simulink model "SRM"  (R2025a)
settings: Solver=VariableStepAuto  StartTime=0.0  StopTime=2.00  RelTol=1e-3
values from neighbouring files (symbols this model uses):
  B = 0.001    [CODE.m]    (also in Controller.m = 0.0001; Moedl.m = Bmat; srm_mpc_setup.m = Bmat)
  Bp1_Current = linspace(0,180,181)    [Lut.m]    (also in Lut_1.m; Lut_Model.m)
  Bp2_Current = linspace(0,0.50,101)    [Lut.m]    (also in Lut_1.m = linspace(0,10,101); Lut_Model.m = linspace(0,10,101))
  J = 0.01    [CODE.m]    (also in Controller.m = 0.001; Lut.m; Moedl.m; srm_mpc_setup.m)
  LuT_Current = zeros(length(Bp1_Current), length(Bp2_Current))    [Lut.m]    (also in Lut_1.m; Lut_Model.m = zeros(181,101))
  Rs = 1    [CODE.m]    (also in Moedl.m; srm_mpc_setup.m)
libraries: spsDiodeLib x6, spsIGBTLib x6, spsVoltageMeasurementLib x3, spsDCVoltageSourceLib x1, sps_lib x1
settings Model: Creator=srima  LastModifiedBy=srima

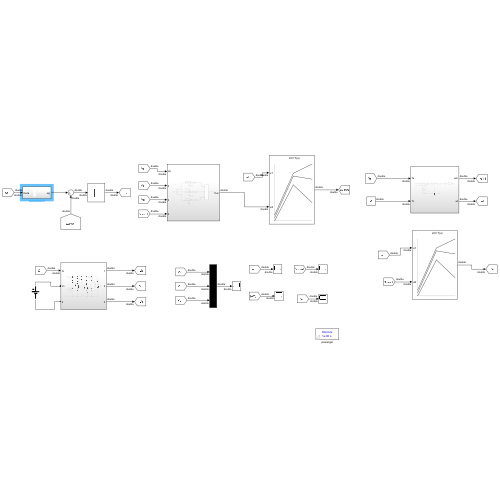
[thumbnail: Simulink's stored preview of the top-level diagram]
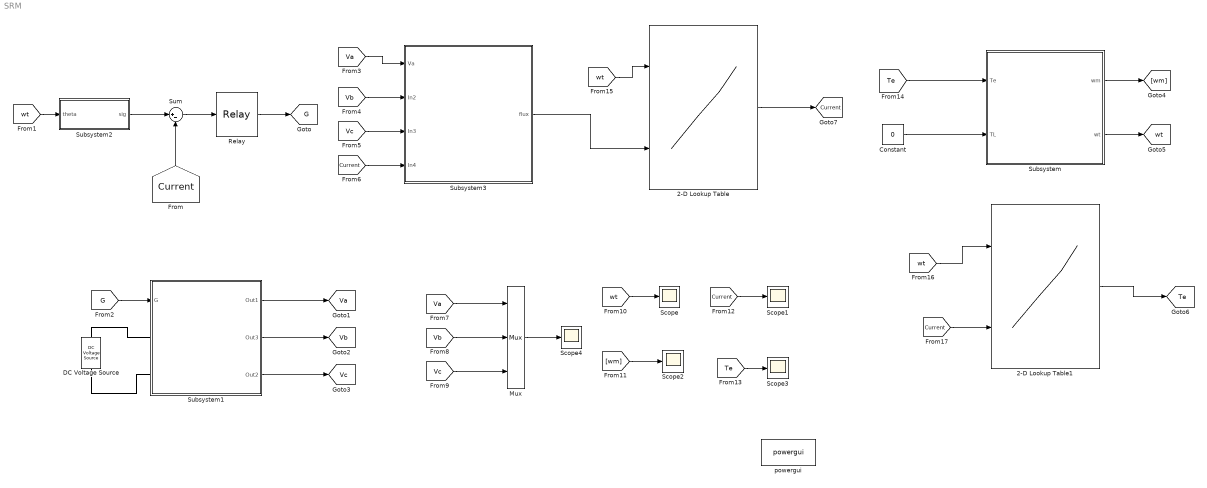
== system SRM ==
  2-D Lookup Table : Lookup_n-D  BreakpointsForDimension1=Bp1_Current  BreakpointsForDimension2=Bp2_Current  Table=LuT_Current  InternalRulePriority=Speed  RndMeth=Simplest
      settings: InputPortMap=u0,u1
  2-D Lookup Table1 : Lookup_n-D  BreakpointsForDimension1=Bp1_Current  BreakpointsForDimension2=Bp2_Current  Table=LuT_Current  InternalRulePriority=Speed  RndMeth=Simplest
      settings: InputPortMap=u0,u1
  Constant : Constant  Value=0
  DC Voltage Source : spsDCVoltageSourceLib/DC Voltage Source  Amplitude=240  Measurements=None
  Mux : Mux  Inputs=3
  Relay : Relay  OnSwitchValue=10  OffSwitchValue=-10
  Scope{,1..4} (5 alike) : Scope
      Scope settings: ActiveDisplayYMinimum=-13.273484846616352  ActiveDisplayYMaximum=186.28058756716342
      Scope1 settings: ActiveDisplayYMinimum=-525.72659240641281  ActiveDisplayYMaximum=1323.506067242982
      Scope2 settings: ActiveDisplayYMinimum=-1.6002807038142943E+8  ActiveDisplayYMaximum=2.6802963440797266E+8  DataLoggingVariableName=ScopeData2
      Scope3 settings: ActiveDisplayYMinimum=41724.804742170025  ActiveDisplayYMaximum=41770.999218996563  DataLoggingVariableName=ScopeData3
      Scope4 settings: ActiveDisplayYMinimum=-1  ActiveDisplayYMaximum=1  DataLoggingVariableName=ScopeData4
  Subsystem : Subsystem
  Subsystem1 : Subsystem
  Subsystem2 : Subsystem
  Subsystem3 : Subsystem
  Sum : Sum  Inputs=|+-
  powergui : sps_lib/powergui  Priority=1  SimulationMode=Discrete  SampleTime=1e-06  frequency=60  Iterations=50  frequencyindice=0  Pbase=100e6  ErrMax=1e-4  UnitsV=kV  UnitsW=MW  buscounter=0  FunctionMessages=off  echomessages=off  EnableUseOfTLC=off  CurrentSourceSwitches=off  DisableSnubberDevices=off  DisableRonSwitches=off  DisableVfSwitches=off  DisplayEquations=off  AutomaticDiscreteSolvers=off  SolverType=Tustin/Backward Euler (TBE)  Interpol=off  ExternalGateDelay=off  methode=off  Ts=100  x0status=blocks  SPID=on  SwTol=0  HookPort=off  NonlinearTolerance=1e-4  nMaxIteration=100  ContinueOnMaxIteration=off  RestoreLinks=warning  ResistiveCurrentMeasurement=off  Frange=[0:2:500]  Ylog=off  Xlog=on  ShowGrid=off  save=off  variable=ZData  structure=0  ZoomFFT=off  StartTime=0.0  cycles=1  DisplayStyle=1  fundamental=60  FreqAxis=off  MaxFrequency=1000  frequencyindicesteady=1  RmsSteady=1  display=off
  tag scope: Current=global, G=global, Te=global, Va=global, Vb=global, Vc=global, wt=global
  wires:
  Sum/1 -> Relay/1
  [Current] -> Sum/2
  Subsystem2/1(sig) -> Sum/1
  [wt] -> Subsystem2/1(theta)
  Relay/1 -> [G]
  Subsystem1/1(Out1) -> [Va]
  Subsystem1/2(Out3) -> [Vb]
  Subsystem1/3(Out2) -> [Vc]
  [G] -> Subsystem1/1(G)
  [Va] -> Subsystem3/1(Va)
  [Vb] -> Subsystem3/2(In2)
  [Vc] -> Subsystem3/3(In3)
  [Current] -> Subsystem3/4(In4)
  [Va] -> Mux/1
  [Vb] -> Mux/2
  [Vc] -> Mux/3
  Mux/1 -> Scope4/1
  [wt] -> Scope/1
  [wm] -> Scope2/1
  [Current] -> Scope1/1
  [Te] -> Scope3/1
  [Te] -> Subsystem/1(Te)
  Constant/1 -> Subsystem/2(TL)
  Subsystem/1(wm) -> [wm]
  Subsystem/2(wt) -> [wt]
  [wt] -> 2-D Lookup Table/1
  Subsystem3/1(flux) -> 2-D Lookup Table/2
  [wt] -> 2-D Lookup Table1/1
  [Current] -> 2-D Lookup Table1/2
  2-D Lookup Table1/1 -> [Te]
  2-D Lookup Table/1 -> [Current]
  connections:
  DC Voltage Source/RConn1 -- Subsystem1/LConn1
  DC Voltage Source/LConn1 -- Subsystem1/LConn2

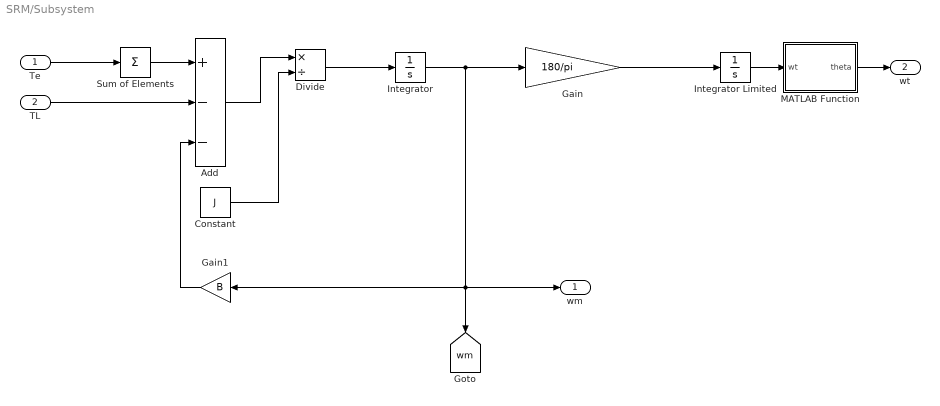
== system SRM/Subsystem ==
  Te : Inport
  TL : Inport  Port=2
  Add : Sum  Inputs=+--
  Constant : Constant  Value=J
  Divide : Product  Inputs=*/
  Gain : Gain  Gain=180/pi
  Gain1 : Gain  Gain=B
  Integrator : Integrator
  Integrator Limited : Integrator  InitialCondition=[0,30,60]  LimitOutput=on
  MATLAB Function : MATLAB Function  TreatAsAtomicUnit=on
  Sum of Elements : Sum  Inputs=+
  wm : Outport
  wt : Outport  Port=2
  tag scope: wm=global
  wires:
  Te/1 -> Sum of Elements/1
  Sum of Elements/1 -> Add/1
  TL/1 -> Add/2
  Gain1/1 -> Add/3
  Divide/1 -> Integrator/1
  Add/1 -> Divide/1
  Constant/1 -> Divide/2
  Gain/1 -> Integrator Limited/1
  Integrator/1 -> wm/1, [wm], Gain1/1, Gain/1
  MATLAB Function/1(theta) -> wt/1
  Integrator Limited/1 -> MATLAB Function/1(wt)

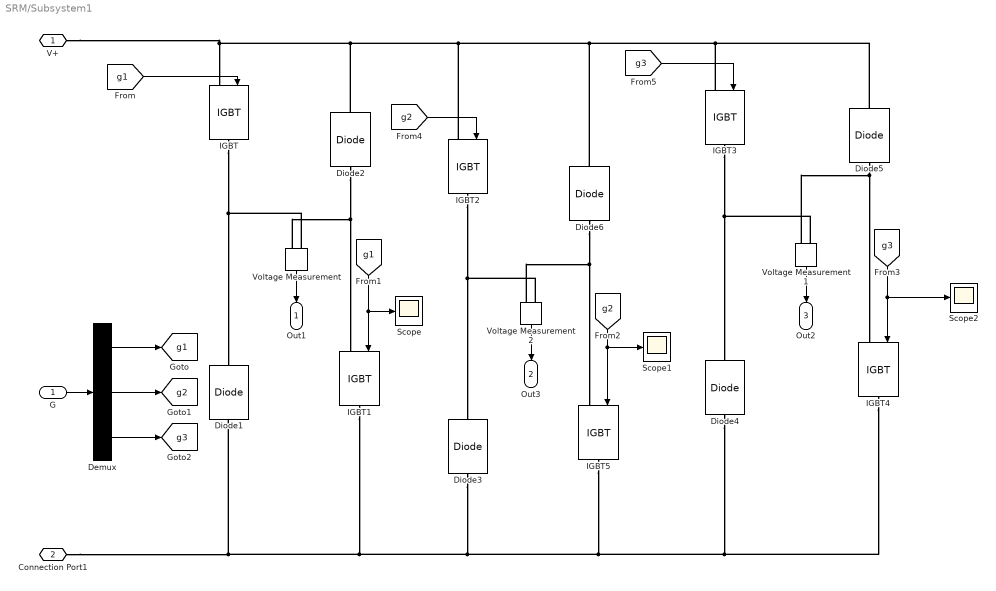
== system SRM/Subsystem1 ==
  G : Inport
  Demux : Demux  Outputs=3
  Diode1 : spsDiodeLib/Diode  Ron=1e-3  Lon=0  Vf=0.8  IC=0  UseSnubber=0  Rs=1000  Cs=inf  Measurements=off
  Diode2 : spsDiodeLib/Diode  Ron=0.001  Lon=0  Vf=0.8  IC=0  UseSnubber=0  Rs=500  Cs=250e-9  Measurements=off
  Diode3 : spsDiodeLib/Diode  Ron=1e-3  Lon=0  Vf=0.8  IC=0  UseSnubber=0  Rs=1000  Cs=inf  Measurements=off
  Diode4 : spsDiodeLib/Diode  Ron=1e-3  Lon=0  Vf=0.8  IC=0  UseSnubber=0  Rs=1000  Cs=inf  Measurements=off
  Diode5 : spsDiodeLib/Diode  Ron=0.001  Lon=0  Vf=0.8  IC=0  UseSnubber=0  Rs=500  Cs=250e-9  Measurements=off
  Diode6 : spsDiodeLib/Diode  Ron=0.001  Lon=0  Vf=0.8  IC=0  UseSnubber=0  Rs=500  Cs=250e-9  Measurements=off
  IGBT{,1..5} (6 alike) : spsIGBTLib/IGBT  Ron=0.001  Lon=0  Vf=1  Tf=1e-6  Tt=2e-6  IC=0  Rs=1e5  Cs=inf  Measurements=off
  Scope : Scope
      settings: ActiveDisplayYMinimum=-0.37134694290744508  ActiveDisplayYMaximum=1.3037726078738059  DataLoggingVariableName=ScopeData5
  Scope1 : Scope
      settings: ActiveDisplayYMinimum=-0.72000513153914225  ActiveDisplayYMaximum=1.7549093677601073  DataLoggingVariableName=ScopeData6
  Scope2 : Scope
      settings: ActiveDisplayYMinimum=-0.70342994389969249  ActiveDisplayYMaximum=5.381855163203106  DataLoggingVariableName=ScopeData7
  Voltage Measurement : spsVoltageMeasurementLib/Voltage Measurement  PhasorSimulation=off  OutputType=Complex  PSBequivalent=0
  Voltage Measurement1 : spsVoltageMeasurementLib/Voltage Measurement  PhasorSimulation=off  OutputType=Complex  PSBequivalent=0
  Voltage Measurement2 : spsVoltageMeasurementLib/Voltage Measurement  PhasorSimulation=off  OutputType=Complex  PSBequivalent=0
  V+ : PMIOPort  Side=Left
  Connection Port1 : PMIOPort  Port=2  Side=Left
  Out1 : Outport
  Out3 : Outport  Port=2
  Out2 : Outport  Port=3
  tag scope: g1=global, g2=global, g3=global
  wires:
  G/1 -> Demux/1
  Demux/1 -> [g1]
  Demux/3 -> [g3]
  Demux/2 -> [g2]
  [g1] -> IGBT/1
  [g1] -> Scope/1, IGBT1/1
  Voltage Measurement/1 -> Out1/1
  Voltage Measurement1/1 -> Out2/1
  [g3] -> IGBT4/1, Scope2/1
  [g2] -> IGBT5/1, Scope1/1
  Voltage Measurement2/1 -> Out3/1
  [g2] -> IGBT2/1
  [g3] -> IGBT3/1
  connections:
  V+/RConn1 -- Diode5/RConn1 -- IGBT3/LConn1 -- Diode6/RConn1 -- IGBT2/LConn1 -- Diode2/RConn1 -- IGBT/LConn1
  IGBT/RConn1 -- Voltage Measurement/LConn1 -- Diode1/RConn1
  Connection Port1/RConn1 -- IGBT4/RConn1 -- Diode4/LConn1 -- IGBT5/RConn1 -- Diode3/LConn1 -- IGBT1/RConn1 -- Diode1/LConn1
  Diode2/LConn1 -- Voltage Measurement/LConn2 -- IGBT1/LConn1
  Diode5/LConn1 -- Voltage Measurement1/LConn2 -- IGBT4/LConn1
  IGBT3/RConn1 -- Voltage Measurement1/LConn1 -- Diode4/RConn1
  IGBT2/RConn1 -- Voltage Measurement2/LConn1 -- Diode3/RConn1
  Diode6/LConn1 -- Voltage Measurement2/LConn2 -- IGBT5/LConn1

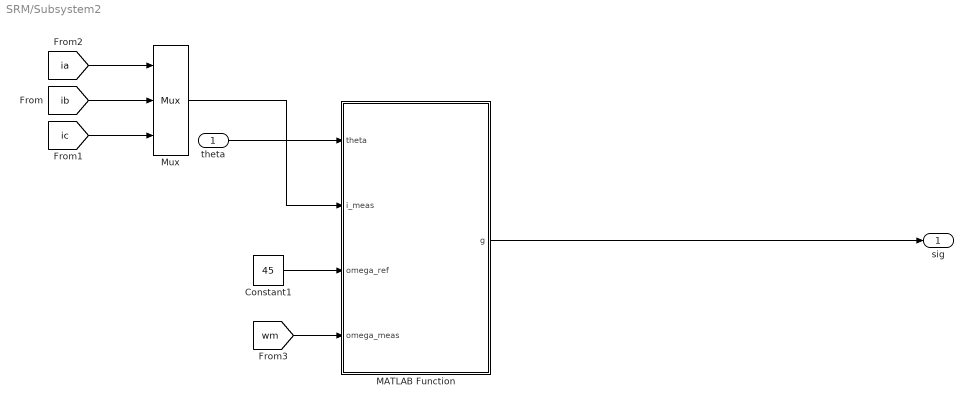
== system SRM/Subsystem2 ==
  theta : Inport
  Constant1 : Constant  Value=45
  MATLAB Function : MATLAB Function  TreatAsAtomicUnit=on
  Mux : Mux  Inputs=3
  sig : Outport
  wires:
  MATLAB Function/1(g) -> sig/1
  theta/1 -> MATLAB Function/1(theta)
  [ia] -> Mux/1
  [ib] -> Mux/2
  [ic] -> Mux/3
  Mux/1 -> MATLAB Function/2(i_meas)
  Constant1/1 -> MATLAB Function/3(omega_ref)
  [wm] -> MATLAB Function/4(omega_meas)

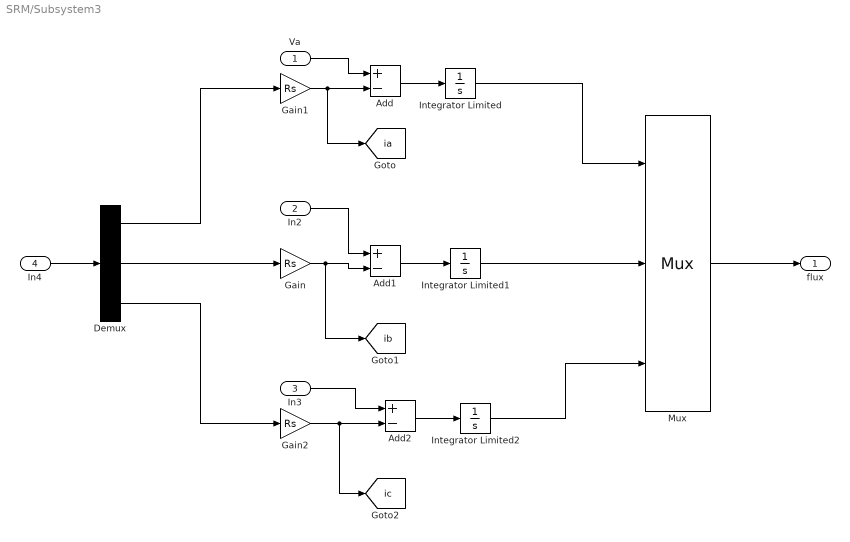
== system SRM/Subsystem3 ==
  Va : Inport
  In2 : Inport  Port=2
  In3 : Inport  Port=3
  In4 : Inport  Port=4
  Add : Sum  Inputs=+-
  Add1 : Sum  Inputs=+-
  Add2 : Sum  Inputs=+-
  Demux : Demux  Outputs=3
  Gain : Gain  Gain=Rs
  Gain1 : Gain  Gain=Rs
  Gain2 : Gain  Gain=Rs
  Integrator Limited : Integrator  LimitOutput=on  UpperSaturationLimit=1  LowerSaturationLimit=0
  Integrator Limited1 : Integrator  LimitOutput=on  UpperSaturationLimit=1  LowerSaturationLimit=0
  Integrator Limited2 : Integrator  LimitOutput=on  UpperSaturationLimit=1  LowerSaturationLimit=0
  Mux : Mux  Inputs=3
  flux : Outport
  tag scope: ia=global, ib=global, ic=global
  wires:
  In4/1 -> Demux/1
  Demux/1 -> Gain1/1
  Demux/2 -> Gain/1
  Demux/3 -> Gain2/1
  In3/1 -> Add2/1
  Gain2/1 -> [ic], Add2/2
  In2/1 -> Add1/1
  Gain/1 -> [ib], Add1/2
  Gain1/1 -> [ia], Add/2
  Va/1 -> Add/1
  Add2/1 -> Integrator Limited2/1
  Add1/1 -> Integrator Limited1/1
  Add/1 -> Integrator Limited/1
  Integrator Limited/1 -> Mux/1
  Integrator Limited1/1 -> Mux/2
  Integrator Limited2/1 -> Mux/3
  Mux/1 -> flux/1

== matlab function SRM/Subsystem2/MATLAB Function ==
  data: theta input; i_meas input; omega_ref input; omega_meas input; g output
function g = fcn(theta, i_meas, omega_ref, omega_meas)
% MPC Controller for SRM
% Inputs:
%   theta       - [3x1] rotor angles
%   i_meas      - [3x1] measured phase currents
%   omega_ref   - scalar speed reference
%   omega_meas  - scalar measured speed
%
% Output:
%   g           - [3x1] gate signals (0 or 1)

% Motor parameters
J  = 0.01;      % inertia
B  = 0.001;     % friction
Kt = 0.2;       % torque constant
Rs = 1;         % resistance
L  = 0.05;      % inductance
Ts = 1e-4;      % sample time

% MPC weights
Np = 3;         % prediction horizon
Q  = 10;        % speed tracking weight
R  = 0.1;       % effort penalty

% Candidate voltages (3 options per phase)
Vdc = 240;
candidates = [0, Vdc, -Vdc];

% Initialize best cost and output
best_cost = inf;
best_g = zeros(3,1);   % numeric [3x1], not logical

% Try all switching combinations
for u1 = candidates
    for u2 = candidates
        for u3 = candidates
            omega_pred = omega_meas;
            i_pred = i_meas;   % [3x1]
            cost = 0;

            for p = 1:Np
                torque = Kt * sum(i_pred);
                omega_pred = omega_pred + Ts*((torque - B*omega_pred)/J);
                i_pred = i_pred + Ts*(([u1; u2; u3] - Rs*i_pred)/L);

                % stage cost
                cost = cost + Q*(omega_ref - omega_pred)^2 ...
                           + R*(u1^2 + u2^2 + u3^2);
            end

            % Check if better
            if cost < best_cost
                best_cost = cost;
                % convert switching decision to [0/1]
                best_g = double([u1 > 0; u2 > 0; u3 > 0]);
            end
        end
    end
end

% Final gate signals
g = best_g;

end

== matlab function SRM/Subsystem/MATLAB Function ==
  data: wt input; theta output
function theta = fcn(wt)

theta = mod(wt,90);
